simulink model "simple_example_extended"  (R2021a)
settings: Solver=VariableStepAuto  StartTime=0.0  StopTime=20  MaxStep=0.01  RelTol=1e-13
libraries: adrc_toolbox_library x1, simulink x1
settings Model: Creator=krzys  LastModifiedBy=PC
settings SolverCC: AlgebraicLoopSolver=TrustRegion
settings DebuggingCC: ArithmeticOperatorsInVariantConditions=warning
settings SFSimCC: CustomCodeUndefinedFunction=UseInterfaceOnly

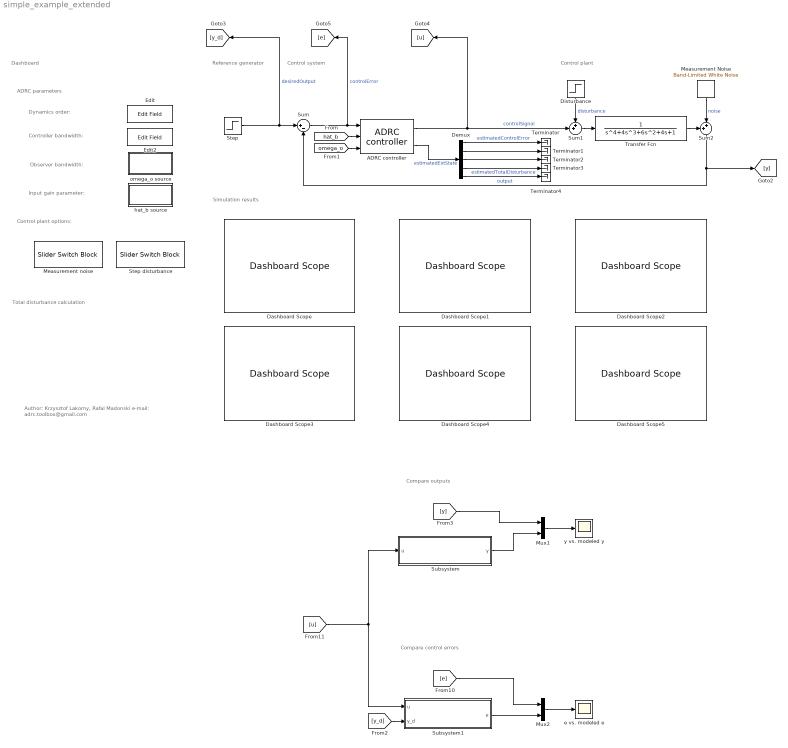
== system simple_example_extended ==
  note: Compare control errors
  note: Compare outputs
  note: Total disturbance calculation
  note: Control plant options:
  note: ADRC parameters
  note: Observer bandwidth:
  note: Controller bandwidth:
  note: Input gain parameter:
  note: Dynamics order:
  note: Dashboard
  note: Simulation results
  note: Reference
      | generator
  note: Control system
  note: Control plant
  note: Author: Krzysztof Lakomy, Rafal Madonski
      | e-mail: adrc.toolbox@gmail.com
  ADRC controller : adrc_toolbox_library/ADRC controller  dynamicsOrder=4  inputGainParameter=0.8  inputGainSource=External  observerBandwidth=50  observerBandwidthSource=External  controllerBandwidth=5  controllerBandwidthSource=Internal  saturationEnabled=on  UpperLimit=100  LowerLimit=-100  deadTimeEnabled=off  deadTime=0.2  observerOutputEnabled=on  observerOutputChoice=Estimated extended state
      settings: SourceProductName=ADRC Toolbox
  Dashboard Scope{,1,3..5} (5 alike) : DashboardScope
  Dashboard Scope2 : DashboardScope  Ymin=-0.10000000000000001  Ymax=0.10000000000000001
  Demux : Demux  Outputs=5
  Disturbance : Step  Time=10  After=0  SampleTime=0
  Edit : EditField  LabelPosition=Hide  ShowInitialText=on  Alignment=Center
  Edit2 : EditField  LabelPosition=Hide  ShowInitialText=on  Alignment=Center
  Measurement Noise : simulink/Sources/Band-Limited White Noise  Cov=0  Ts=0.01  seed=[23341]
  Measurement noise : SliderSwitchBlock  LabelPosition=Hide
      settings: Values={{'Off', 'On'}, [0 1e-14]}
  Mux1 : Mux  Inputs=2
  Mux2 : Mux  Inputs=2
  Step : Step  After=15  SampleTime=0
  Step disturbance : SliderSwitchBlock  LabelPosition=Hide
      settings: Values={{'Off', 'On'}, [0 70]}
  Subsystem : Subsystem
  Subsystem1 : Subsystem
  Sum : Sum  Inputs=|+-
  Sum1 : Sum  Inputs=++|
  Sum2 : Sum  Inputs=++|
  Terminator{,1..4} (5 alike) : Terminator
  Transfer Fcn : TransferFcn  Denominator=[1 4 6 4 1]
  e vs. modeled e : Scope
  hat_b source : Subsystem
  omega_o source : Subsystem
  y vs. modeled y : Scope
  wires:
  Sum/1 -> [e], ADRC controller/1  "controlError"
  Transfer Fcn/1 -> Sum2/1
  Sum1/1 -> Transfer Fcn/1
  Disturbance/1 -> Sum1/1  "disturbance"
  ADRC controller/1 -> [u], Sum1/2  "controlSignal"
  Sum2/1 -> [y], Sum/2  "output"
  Measurement Noise/1 -> Sum2/2  "noise"
  Step/1 -> [y_d], Sum/1  "desiredOutput"
  ADRC controller/2 -> Demux/1  "estimatedExtState"
  Demux/1 -> Terminator/1  "estimatedControlError"
  Demux/2 -> Terminator1/1
  Demux/3 -> Terminator2/1
  Demux/4 -> Terminator3/1
  Demux/5 -> Terminator4/1  "estimatedTotalDisturbance"
  [hat_b] -> ADRC controller/2
  [omega_o] -> ADRC controller/3
  Mux2/1 -> e vs. modeled e/1
  [u] -> Subsystem/1(u), Subsystem1/1(u)
  [y_d] -> Subsystem1/2(y_d)
  Subsystem/1(y) -> Mux1/2
  Mux1/1 -> y vs. modeled y/1
  [e] -> Mux2/1
  Subsystem1/1(e) -> Mux2/2
  [y] -> Mux1/1

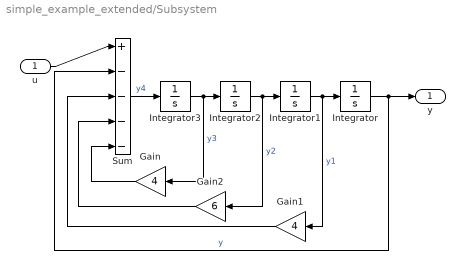
== system simple_example_extended/Subsystem ==
  u : Inport
  Gain : Gain  Gain=4
  Gain1 : Gain  Gain=4
  Gain2 : Gain  Gain=6
  Integrator{,1..3} (4 alike) : Integrator
  Sum : Sum  Inputs=|+----
  y : Outport
  wires:
  u/1 -> Sum/1
  Integrator/1 -> Sum/2, y/1  "y"
  Integrator1/1 -> Gain1/1, Integrator/1  "y1"
  Integrator2/1 -> Gain2/1, Integrator1/1  "y2"
  Integrator3/1 -> Gain/1, Integrator2/1  "y3"
  Sum/1 -> Integrator3/1  "y4"
  Gain/1 -> Sum/5
  Gain1/1 -> Sum/3
  Gain2/1 -> Sum/4

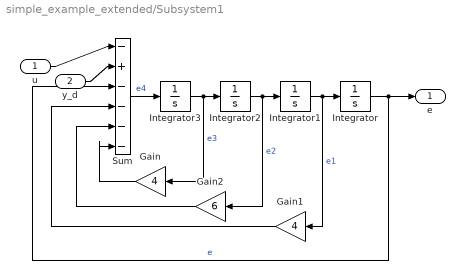
== system simple_example_extended/Subsystem1 ==
  u : Inport
  y_d : Inport  Port=2
  Gain : Gain  Gain=4
  Gain1 : Gain  Gain=4
  Gain2 : Gain  Gain=6
  Integrator{,1..3} (4 alike) : Integrator
  Sum : Sum  Inputs=|-+----
  e : Outport
  wires:
  Gain2/1 -> Sum/5
  Gain1/1 -> Sum/4
  Gain/1 -> Sum/6
  Sum/1 -> Integrator3/1  "e4"
  Integrator3/1 -> Integrator2/1, Gain/1  "e3"
  Integrator2/1 -> Integrator1/1, Gain2/1  "e2"
  Integrator1/1 -> Integrator/1, Gain1/1  "e1"
  Integrator/1 -> Sum/3, e/1  "e"
  u/1 -> Sum/1
  y_d/1 -> Sum/2

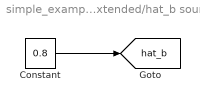
== system simple_example_extended/hat_b source ==
  Constant : Constant  Value=0.8
  tag scope: hat_b=global
  wires:
  Constant/1 -> [hat_b]

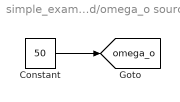
== system simple_example_extended/omega_o source ==
  Constant : Constant  Value=50
  tag scope: omega_o=global
  wires:
  Constant/1 -> [omega_o]
